simulink model "c2407cantest"  (Simulink 6.0)
settings: Solver=FixedStepDiscrete  SolverMode=SingleTasking  StartTime=0.0  StopTime=inf  RelTol=1e-3
libraries: c2400dspchiplib x3, c2000tgtpreflib x1, memblks x1
settings Model: Creator=zgalijas  LastModifiedBy=zgalijas  ProdHWDeviceType=TI C2000
settings DataIOCC: SaveOutput=off  SaveTime=off  SignalLoggingName=sigsOut
settings OptimizationCC: InlineInvariantSignals=off
settings DebuggingCC: CheckExecutionContextPreStartOutputMsg=on  CheckExecutionContextRuntimeOutputMsg=on  SolverPrmCheckMsg=none
settings HardwareCC: ProdBitPerChar=16  ProdBitPerInt=16  ProdIntDivRoundTo=Zero  ProdEndianess=LittleEndian  ProdWordSize=16  ProdHWDeviceType=TI C2000  TargetHWDeviceType=32-bit Generic
settings ModelReferenceCC: UpdateModelReferenceTargets=IfOutOfDate
settings RTWCC: SystemTargetFile=ti_c2000_grt.tlc  GenCodeOnly=on  TemplateMakefile=ti_c2000_grt.tmf  ProcessScript=ti_c2000_grt_make_rtw_hook
settings STFCustomTargetCC: TargetFcnLib=ansi_tfl_tmw.mat  GenFloatMathFcnCalls=ANSI_C  ModelReferenceCompliant=off  SystemTargetFile=ti_c2000_grt.tlc  ActivateCallback=ti_c2000_callback('ActivateCallback',hSrc,hDlg);  ForcedBaseTarget=off
settings GRTTargetCC: ModelReferenceCompliant=off  MatFileLogging=off
settings SFSimCC: SFSimApplyToAllLibs=on  SFSimBuildMode=Incremental

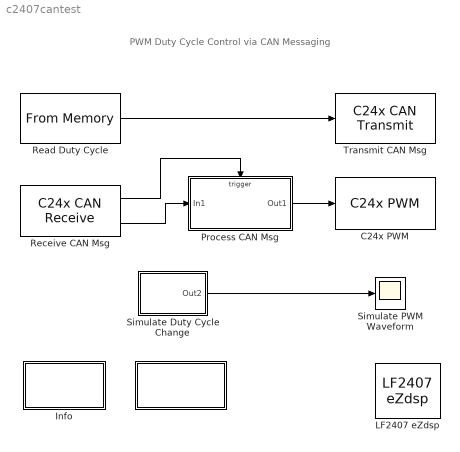
== system c2407cantest ==
  note: PWM Duty Cycle Control via CAN Messaging
  " " : Subsystem  PropExecContextAcrossSSBoundary=on
      settings: OpenFcn=runc2xxxcantest
      mask Type: Run demo
      mask Display: disp(sprintf('Build/Reload\n& Run'))
  " Info" : Subsystem  PropExecContextAcrossSSBoundary=on
      mask Display: disp('Info')
  C24x PWM : c2400dspchiplib/C24x PWM  useModule=A  timerSource=Specify via dialog  timerPeriod=64000  waveformType=Symmetric  unit1Status=on  unit1Source=Input port  unit1Value=2000  unit2Status=off  unit2Source=Input port  unit2Value=2000  unit3Status=off  unit3Source=Input port  unit3Value=2000  unit1_1Logic=Active low  unit1_2Logic=Active high  unit2_1Logic=Active high  unit2_2Logic=Active low  unit3_1Logic=Active high  unit3_2Logic=Active low  enableDeadband1=off  enableDeadband2=off  enableDeadband3=off  deadbandPrescaler=1  deadbandPeriod=1  adcstartEvent=None
  LF2407 eZdsp : c2000tgtpreflib/LF2407 eZdsp  Tag=C2000 TARGET PREFERENCES BLOCK
  Process CAN Msg : Subsystem  Tag=20  TreatAsAtomicUnit=on  PropExecContextAcrossSSBoundary=on
  Read Duty Cycle : memblks/From Memory  Tag=5  memAddressMask=8FF0  dType=uint16  Ts=1/10  frameSize=1
  Receive CAN Msg : c2400dspchiplib/C24x CAN Receive  Tag=15  mailboxNo=0  messageID=bin2dec('111000111')  messageType=Standard (11-bit identifier)  sampleTime=1/10  dataType=uint16  outputMessageLength=off  outputMessageTimeStamp=off
  Simulate PWM Waveform : Scope
      settings: TimeRange=10  YMin=0  YMax=17500  MaxDataPoints=10000
  Simulate Duty Cycle Change : Subsystem  PropExecContextAcrossSSBoundary=on  mask{dutyCycle=75 %}
      mask prompts: dutyCycle "Duty Cycle"
      mask StyleString: popup(25 %|50 %|75 %)
      mask Display: disp ('Duty Cycle\nChange')
  Transmit CAN Msg : c2400dspchiplib/C24x CAN Transmit  Tag=10  mailboxNo=5  messageID=bin2dec('111000111')  messageType=Standard (11-bit identifier)
  wires:
  Read Duty Cycle/1 -> Transmit CAN Msg/1
  Receive CAN Msg/2 -> Process CAN Msg/1(In1)
  Receive CAN Msg/1 -> Process CAN Msg/Trigger
  Simulate Duty Cycle Change/1(Out2) -> Simulate PWM Waveform/1
  Process CAN Msg/1(Out1) -> C24x PWM/1

== system c2407cantest/  ==

== system c2407cantest/ Info ==
  note: This example demonstrates the use of the c2407 CAN Receive, c2407 CAN Transmit,
      | C2407 PWM, and C2407 From Memory blocks in generating the pulse waveform.
      |
      | "Read Duty Cycle" reads duty cycle value stored at the memory location 0xFFE0. This value
      | controls the width of the pulse waveform generated by the PWM1 while its period is fixed at
      | 64000 clock cycles.
      |
      | "Transmit CAN Msg" uses mailbox 5 to transmit duty cycle value packed in a standard CAN
      | message frame, while "Receive CAN Msg" uses mailbox 0 to receive it.
      |
      | "Process CAN Msg" unpacks the duty cycle value and sends it to the PWM. The duty cycle of
      | the generated pulse waveform is determined by the relative ratio of the pulse width and the
      | pulse period. In this example, the duty cycle toggles between 25%, 50%, and 75% based on
      | users selection. This effect can be observed on the oscilloscope.
      |
      | PWM Duty Cycle can be changed while the generated code is running using "write" method
      | of the companion product Link for Code Composer Studio. Select either 25%, 50%, or 75%
      | value from the GUI that opens up when "Build/Reload & Run" is pressed.
      |
      | "Simulate Duty Cycle Change" and "Simulate PWM Waveform" are dedicated to simulation
      | only. Use these blocks to simulate and observe effects achieved with the generated code.
  note: The code generation portion of this demo requires the following hardware:
      |
      | Spectrum Digital eZdsp LF2407
      | Oscilloscope and probes
      |
      | Connect the output of PWM1 on the eZdsp LF2407 to the analog input of the oscilloscope.
  note: Setup:
  note: Demo Description:

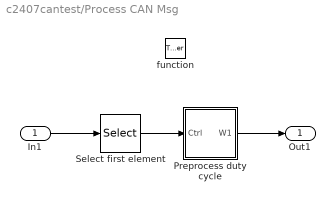
== system c2407cantest/Process CAN Msg ==
  In1 : Inport  LatchInput=off
  function : TriggerPort  TriggerType=function-call
  Preprocess duty cycle : Subsystem  Tag=30  PropExecContextAcrossSSBoundary=on
  Select first element : Selector  Elements=[1]  InputPortWidth=4
  Out1 : Outport
  wires:
  In1/1 -> Select first element/1
  Preprocess duty cycle/1(W1) -> Out1/1
  Select first element/1 -> Preprocess duty cycle/1(Ctrl)

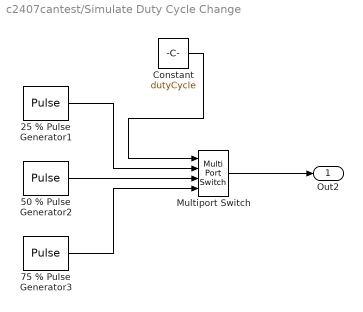
== system c2407cantest/Simulate Duty Cycle Change ==
  25 % Pulse Generator1 : DiscretePulseGenerator  Amplitude=16000  Period=4000  PulseWidth=1000  SampleTime=64/80000
  50 % Pulse Generator2 : DiscretePulseGenerator  Amplitude=16000  Period=4000  PulseWidth=2000  SampleTime=64/80000
  75 % Pulse Generator3 : DiscretePulseGenerator  Amplitude=16000  Period=4000  PulseWidth=3000  SampleTime=64/80000
  Constant : Constant  Value=dutyCycle
  Multiport Switch : MultiPortSwitch  Inputs=3  SaturateOnIntegerOverflow=on
  Out2 : Outport
  wires:
  Multiport Switch/1 -> Out2/1
  75 % Pulse Generator3/1 -> Multiport Switch/4
  Constant/1 -> Multiport Switch/1
  25 % Pulse Generator1/1 -> Multiport Switch/2
  50 % Pulse Generator2/1 -> Multiport Switch/3

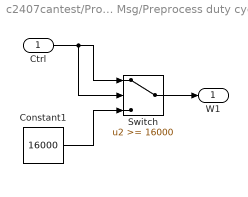
== system c2407cantest/Process CAN Msg/Preprocess duty cycle ==
  Ctrl : Inport  LatchInput=off
  Constant1 : Constant  Tag=31  Value=16000  OutDataTypeMode=uint16
  Switch : Switch  Tag=32  Threshold=16000  ZeroCross=off
  W1 : Outport
  wires:
  Constant1/1 -> Switch/3
  Ctrl/1 -> Switch/2, Switch/1
  Switch/1 -> W1/1
